simulink model "dsa2k_iwave_ospfb_4800"  (R2021a)
settings: Solver=VariableStepAuto  StartTime=0.0  StopTime=10.0  RelTol=1e-3
undefined symbols (not defined in the file): datetime, i, posixtime
libraries: xbsIndex_r4 x6279, casper_library_misc x96, casper_library_reorder x16, casper_library_delays x16, casper_library_accumulators x7, xps_library x3
(part 1 of 75)
settings Model: Creator=jackh  LastModifiedBy=jackh

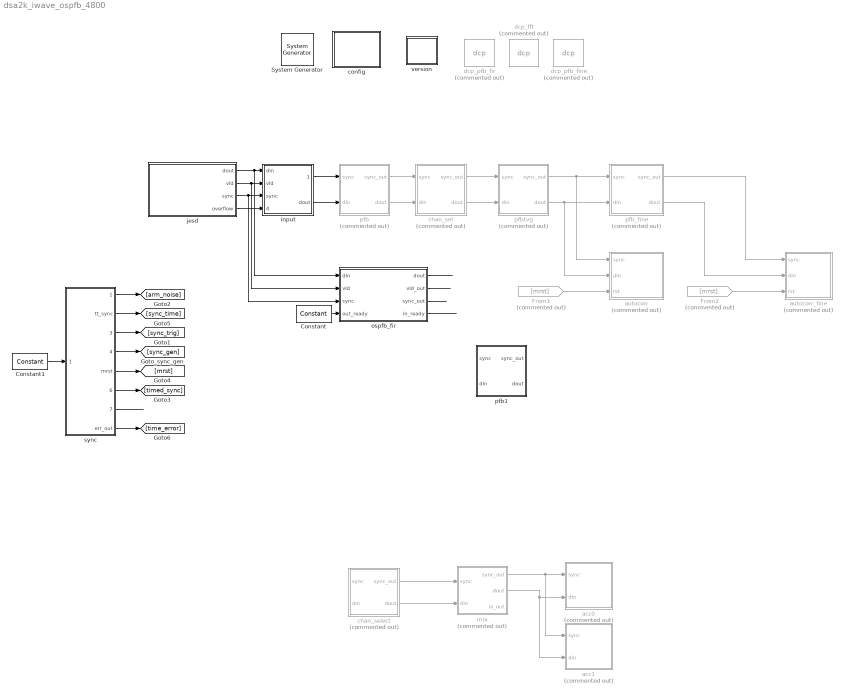
== system dsa2k_iwave_ospfb_4800 ==
  " System Generator" : xbsIndex_r4/ System Generator  Tag=genX  xilinxfamily=zynquplus  part=xczu11eg  speed=-1-i  package=ffvc1760  synthesis_tool=XST  clock_wrapper=Clock Enables  directory=/home/jackh/src/dsa2000-fpga/firmware/src/models/dsa2k_iwave_ospfb_4800/sysgen  proj_type=Vivado  Synth_file=Vivado Synthesis Defaults  Impl_file=Vivado Implementation Defaults  testbench=off  simulink_period=1  sysclk_period=3.3333  dcm_input_clock_period=10  incr_netlist=off  trim_vbits=Everywhere in SubSystem  dbl_ovrd=According to Block Masks  core_generation=According to Block Masks  run_coregen=off  deprecated_control=off  eval_field=0  block_type=sysgen
  Constant : xbsIndex_r4/Constant  const=1.0  gui_display_data_type=Boolean  arith_type=Boolean  n_bits=16  bin_pt=14  preci_type=Single  exp_width=8  frac_width=24  explicit_period=on  period=1  equ=P=C  opselect=C  inp2=PCIN>>17  opr=+  inp1=P  carry=CIN  dbl_ovrd=off  block_type=constant
  Constant1 : xbsIndex_r4/Constant  const=0  gui_display_data_type=Boolean  arith_type=Boolean  n_bits=16  bin_pt=14  preci_type=Single  exp_width=8  frac_width=24  explicit_period=on  period=1  equ=P=C  opselect=C  inp2=PCIN>>17  opr=+  inp1=P  carry=CIN  dbl_ovrd=off  block_type=constant
  From1 : From  Commented=on  GotoTag=mrst
  From2 : From  Commented=on  GotoTag=mrst
  acc0 : Subsystem  Commented=on  mask{nchan_serial_bits=8}
      mask prompts: nchan_serial_bits "Number of serial channels (2^?)"
  acc1 : Subsystem  Commented=on  mask{nchan_serial_bits=8}
      mask prompts: nchan_serial_bits "Number of serial channels (2^?)"
  autocorr : Subsystem  Commented=on  mask{nchan_bits=10-3, npol_bits=0}
      mask prompts: nchan_bits "Number of *SERIAL* channels (2^?)"; npol_bits "Number of pols (2^?)"
  autocorr_fine : Subsystem  Commented=on  mask{nchan_bits=14-3, npol_bits=0}
      mask prompts: nchan_bits "Number of *SERIAL* channels (2^?)"; npol_bits "Number of pols (2^?)"
  chan_sel : Subsystem  Commented=on
  chan_select : Subsystem  Commented=on  mask{serial_chan_bits=8}
      mask prompts: serial_chan_bits "Number of serial channels (2^?)"
  config : Subsystem  Tag=xps:xsg  mask(xsg core config){hw_sys=iwave_zu11:xczu11eg, clk_src=dsp_clk, clk_rate=4800/16 * 4 / 3, no_block_diagram=on, sample_period=1, synthesis_tool=XST}
      mask prompts: hw_sys "Hardware Platform"; clk_src "User IP Clock source"; clk_rate "User IP Clock Rate (MHz)"; no_block_diagram "Skip inclusion of infrastructure block diagram"; sample_period "Sample Period"; synthesis_tool "Synthesis Tool:"
      mask help:
      | The XSG Core Config block is used to configure the System Generator design
      | for the casper_xps toolflow. Settings here are used to configure the
      | Xilinx System Generator block parameters automatically, and control toolflow
      | script  execution. It needs to be at the top level of all designs being compiled
      | with the casper_xps toolflow.
      mask init:
      | xps_xsg_iwave_zu11_conf_mask;
      mask Help: eval('xlWeb([getenv(''MLIB_ROOT''), ''\doc\html\sys_xsg_core_config\sys_xsg_core_config.html''])')
      mask TypeOptions hw_sys: iwave_zu11:xczu11eg
      mask TypeOptions clk_src: sys_clk | adc_clk | clk300mhz | dsp_clk
      mask TypeOptions synthesis_tool: Leonardo Spectrum | Synplify | Synplify Pro | XST
      mask Display: fprintf(['iWave_ZU11']);
  dcp_fft : xps_library/Utilities/dcp  Tag=xps:dcp  Commented=on  dcp_file=[fileparts(which(bdroot)) '/dsp/fft_2p_4kc_18i_18o_core/fft_2p_4kc_18i_18o_core.dcp']
      settings: SourceProductName=CASPER XPS Blockset
  dcp_pfb_fine : xps_library/Utilities/dcp  Tag=xps:dcp  Commented=on  dcp_file=[fileparts(which(bdroot)) '/dsp/pfb_fine_core/pfb_fine_core.dcp']
      settings: SourceProductName=CASPER XPS Blockset
  dcp_pfb_fir : xps_library/Utilities/dcp  Tag=xps:dcp  Commented=on  dcp_file=[fileparts(which(bdroot)) '/dsp/pfb_fir_2p_2kpt_12i_18o_os2_core/pfb_fir_2p_2kpt_12i_18o_os2_core.dcp']
      settings: SourceProductName=CASPER XPS Blockset
  input : Subsystem
  jesd : Subsystem  Tag=xps:adi_jesd  mask(xsg_adi_jesd){fmc_port=0, adi_ip_path=/home/jackh/src/dsa2000-fpga/firmware/lib/adi_hdl/library, sample_rate_mhz=4800}
      mask prompts: fmc_port "FMC Port Number"; adi_ip_path "Path to ADI IP repository"; sample_rate_mhz "Sample rate (Msps)"
      mask init:
      | adi_jesd_init()
      mask Help: eval('xlWeb([getenv(''MLIB_ROOT''), ''\doc\html\sys_xsg_core_config\sys_xsg_core_config.html''])')
  mix : Subsystem  Commented=on  mask{serial_chan_bits=8}
      mask prompts: serial_chan_bits "Number of serial channels (2^?)"
  ospfb_fir : Subsystem  Tag=xps:ospfb_fir  mask(xsg_ospfb_fir){constants_path=[fileparts(which(bdroot)) '/config'], coeffs_path=[fileparts(which(bdroot)) '/config'], samples_per_clock=16}
      mask prompts: constants_path "Directory containing alpaca_constants_pkg.sv"; coeffs_path "Directory containing alpaca_ospfb_hann_2048_8_coeff_pkg.sv"; samples_per_clock "Parallel samples per clock"
      mask init:
      | ospfb_fir_init()
      mask Help: eval('xlWeb([getenv(''MLIB_ROOT''), ''\doc\html\sys_xsg_core_config\sys_xsg_core_config.html''])')
  pfb : Subsystem  Commented=on
  pfb1 : Subsystem
  pfb_fine : Subsystem  Commented=on
  pfbtvg : Subsystem  Commented=on  mask{serial_chan_bits=8}
      mask prompts: serial_chan_bits "Serial channels (2^?)"
  sync : Subsystem  mask{sync_lsb_bits=14, sync_period=12800000}
      mask prompts: sync_lsb_bits "Allowed sync granularity (2^?)"; sync_period "Expected_sync_period"
  version : Subsystem  mask{fw_type=2, ver_maj=1, ver_min=0, ver_rev=0, ver_bugfix=0}
      mask prompts: fw_type "Firmware Type"; ver_maj "Major version"; ver_min "Minor version"; ver_rev "Revision"; ver_bugfix "Bugfix"
  wires:
  sync/1(arm_noise) -> [arm_noise]
  sync/2(tt_sync) -> [sync_time]
  sync/5(mrst) -> [mrst]
  sync/3(ext_sync) -> [sync_trig]
  sync/6(timed_sync) -> [timed_sync]
  sync/4(sync_out) -> [sync_gen]
  sync/8(err_out) -> [time_error]
  sync/7(tt_int_out) -> ?
  Constant1/1 -> sync/1(sync_in)
  input/1(sync_out) -> pfb/1(sync)
  input/2(dout) -> pfb/2(din)
  pfbtvg/1(sync_out) -> pfb_fine/1(sync), autocorr/1(sync)
  chan_select/1(sync_out) -> mix/1(sync)
  chan_select/2(dout) -> mix/2(din)
  mix/1(sync_out) -> acc1/1(sync), acc0/1(sync)
  mix/2(dout) -> acc1/2(din), acc0/2(din)
  From1/1 -> autocorr/3(rst)
  jesd/2(vld) -> ospfb_fir/2(vld), input/2(vld)
  jesd/3(sync) -> ospfb_fir/3(sync), input/3(sync)
  jesd/4(overflow) -> input/4(overflow)
  jesd/1(dout) -> ospfb_fir/1(din), input/1(din)
  pfbtvg/2(dout) -> pfb_fine/2(din), autocorr/2(din)
  pfb_fine/2(dout) -> autocorr_fine/2(din)
  From2/1 -> autocorr_fine/3(rst)
  pfb_fine/1(sync_out) -> autocorr_fine/1(sync)
  pfb/1(sync_out) -> chan_sel/1(sync)
  pfb/2(dout) -> chan_sel/2(din)
  chan_sel/1(sync_out) -> pfbtvg/1(sync)
  chan_sel/2(dout) -> pfbtvg/2(din)
  Constant/1 -> ospfb_fir/4(out_ready)
  ospfb_fir/1(dout) -> ?
  ospfb_fir/2(vld_out) -> ?
  ospfb_fir/3(sync_out) -> ?
  ospfb_fir/4(in_ready) -> ?

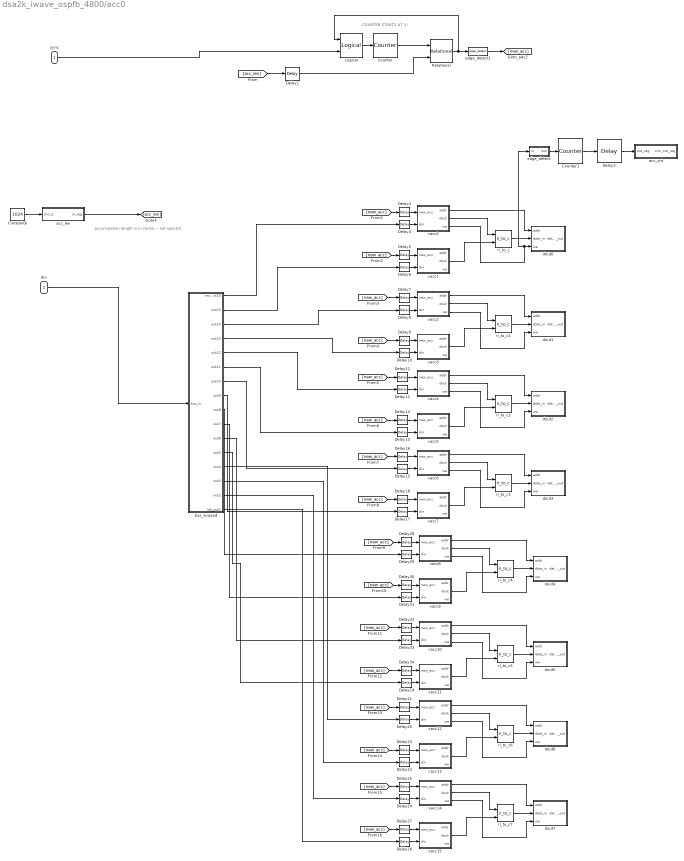
== system dsa2k_iwave_ospfb_4800/acc0 ==
  note: COUNTER STARTS AT 1!
  note: accumulation length is in clocks -- not spectra
  sync : Inport
  din : Inport  Port=2
  Constant6 : Constant  Value=1024
  Counter : xbsIndex_r4/Counter  cnt_type=Free Running  cnt_to=Inf  operation=Up  start_count=1  cnt_by_val=1  arith_type=Unsigned  n_bits=32  bin_pt=0  load_pin=off  rst=on  en=off  explicit_period=on  period=1  use_behavioral_HDL=on  implementation=Fabric  dbl_ovrd=off  block_type=counter
  Counter1 : xbsIndex_r4/Counter  cnt_type=Free Running  cnt_to=Inf  operation=Up  start_count=0  cnt_by_val=1  arith_type=Unsigned  n_bits=32  bin_pt=0  load_pin=off  rst=off  en=on  explicit_period=on  period=1  use_behavioral_HDL=on  implementation=Fabric  dbl_ovrd=off  block_type=counter
  Delay{1..34} (34 alike) : xbsIndex_r4/Delay  rst=off  infoeditControl=Selection of Reset will increase slice count due to use of real FFs and instead of SRLs  en=off  latency=1  reg_retiming=on  dbl_ovrd=off  block_type=delay
  Logical : xbsIndex_r4/Logical  logical_function=OR  inputs=2  en=off  latency=0  precision=Full  arith_type=Unsigned  n_bits=16  bin_pt=0  align_bp=on  dbl_ovrd=off  block_type=logical
  Relational : xbsIndex_r4/Relational  mode=a=b  op_type=Bool  en=off  latency=0  dbl_ovrd=off  block_type=relational
  acc_cnt : Subsystem  Tag=xps:sw_reg  AncestorBlock=xps_library/Memory/software_register  mask(swreg){io_dir=To Processor, io_delay=0, init_val=0, sample_period=1, names=reg, bitwidths=32, bin_pts=0, arith_types=0, sim_port=on, show_format=on, desc_str=|}
      mask desc_str=|
      | 32-bit wrapping accumulation counter, which increments each
      | time a new accumulation is recorded to RAM.
      | There is no buffer locking when correlation data are
      | read, so this counter can be used to ensure that data
      | have not changed during a read.
      mask prompts: io_dir "I/O direction"; io_delay "I/O delay"; init_val "Initial Value"; sample_period "Sample period"; names "Bitfield names [msb...lsb]"; bitwidths "Bitfield widths"; bin_pts "Bitfield binary pts"; arith_types "Bitfield types, ufix=0, fix=1, bool=2"; sim_port "Provide sim input/output?"; show_format "Print format string?"; desc_str "Description"
      mask help: A 32-bit software-accessible register. Can be divided into bitfields of varying widths and types using the fields in the block mask.
      mask init:
      | swreg_init(gcb)
      settings: AttributesFormatString=1output:uf32.0 = 32 bits
      mask TypeOptions io_dir: To Processor | From Processor
      mask Callback io_dir:
      | mask_enables = get_param(gcb, 'MaskEnables');
      | mask_names = get_param(gcb, 'MaskNames');
      | if strcmp(get_param(gcb, 'io_dir'), 'To Processor'),
      |     mask_enables{ismember(mask_names, 'sample_period')} = 'off';
      | else
      |     mask_enables{ismember(mask_names, 'sample_period')} = 'on';
      | end
      | set_param(gcb, 'MaskEnables', mask_enables);
      mask DialogControl ParameterTabVar0 Prompt: Setup
  acc_len : Subsystem  Tag=xps:sw_reg  AncestorBlock=xps_library/Memory/software_register  mask(swreg){io_dir=From Processor, io_delay=0, init_val=0, sample_period=1, names=reg, bitwidths=32, bin_pts=0, arith_types=0, sim_port=on, show_format=on, desc_str=|}
      mask desc_str=|
      | Accumulation length, in FPGA clock cycles. To specify
      | an accumulation length as a number of spectra this
      | register should be written with ``number_of_spectra x
      | frequency_channels_per_spectra``. Here the number
      | of frequency channels per spectra is the number
      | *output* by the correlation subsystem.
      | Glitches may occur (resulting in the no new
      | accumulations for a few seconds) if the value in this
      | register is reduced without re-applying a sync to the
      | correlation module.
      mask prompts: io_dir "I/O direction"; io_delay "I/O delay"; init_val "Initial Value"; sample_period "Sample period"; names "Bitfield names [msb...lsb]"; bitwidths "Bitfield widths"; bin_pts "Bitfield binary pts"; arith_types "Bitfield types, ufix=0, fix=1, bool=2"; sim_port "Provide sim input/output?"; show_format "Print format string?"; desc_str "Description"
      mask help: A 32-bit software-accessible register. Can be divided into bitfields of varying widths and types using the fields in the block mask.
      mask init:
      | swreg_init(gcb)
      settings: AttributesFormatString=1input:uf32.0 = 32 bits
      mask TypeOptions io_dir: To Processor | From Processor
      mask Callback io_dir:
      | mask_enables = get_param(gcb, 'MaskEnables');
      | mask_names = get_param(gcb, 'MaskNames');
      | if strcmp(get_param(gcb, 'io_dir'), 'To Processor'),
      |     mask_enables{ismember(mask_names, 'sample_period')} = 'off';
      | else
      |     mask_enables{ismember(mask_names, 'sample_period')} = 'on';
      | end
      | set_param(gcb, 'MaskEnables', mask_enables);
      mask DialogControl ParameterTabVar0 Prompt: Setup
  bus_expand : Subsystem  AncestorBlock=casper_library_flow_control/bus_expand  mask(bus_expand){mode=divisions of equal size, outputNum=16, outputWidth=20, outputBinaryPt=18, outputArithmeticType=1, show_format=off, outputToWorkspace=off, variablePrefix=out, outputToModelAsWell=on}
      mask prompts: outputNum "Number of outputs:"; outputWidth "Output width:"; outputBinaryPt "Output binary point position:"; outputArithmeticType "Output arithmetic type (ufix=0, fix=1, bool=2):"; show_format "Print format string?"; outputToWorkspace "Output to workspace?"; variablePrefix "Variable name prefix:"; outputToModelAsWell "Output to model as well?"
      mask help:
      | Expands a 'bus' made using a bus_create or Xilinx
      | concat block.
      | The input will be divided into the specified number
      | of outputs with the specified arithmetic types.
      | Divisions are made from most significant bit.
      mask init:
      | bus_expand_init(gcb,...
      |     'mode', mode, ...
      |     'outputNum', outputNum, ...
      |     'outputWidth', outputWidth, ...
      |     'outputBinaryPt', outputBinaryPt, ...
      |     'outputArithmeticType', outputArithmeticType, ...
      |     'show_format', show_format, ...
      |     'outputToWorkspace', outputToWorkspace, ...
      |     'variablePrefix', variablePrefix, ...
      |     'outputToModelAsWell', outputToModelAsWell);
      settings: AttributesFormatString=16 outputs
      mask TypeOptions mode: divisions of equal size | divisions of arbitrary size
      mask Callback mode: %bus_expand_callback();
      mask Callback outputWidth: %bus_expand_callback();
      mask Callback outputToWorkspace: %bus_expand_callback();
  dout0 : Subsystem  Tag=xps:bram  AncestorBlock=xps_library/Memory/shared_bram  mask{sample_rate=1, init_vals=[0:2^10-1], data_bin_pt=0, optimization=Minimum_Area, reg_core_output=off, reg_prim_output=off, data_width=64, addr_width=nchan_serial_bits, arith_type=Unsigned, desc_str=|, type_desc=uint64}
      mask desc_str=|
      | Correlation data buffer. Word ``[2n]`` is the
      | real part of the correlation of frequency channel ``n``
      | (after any channel averaging). Word ``[2n+1]`` is
      | the imaginary part of this correlation.
      mask prompts: sample_rate "Sample rate"; init_vals "Initial values (simulation only)"; data_bin_pt "Data Binary Point"; reg_core_output "Register Core Output"; reg_prim_output "Register Primitive Output"; data_width "Data Width"; addr_width "Address width"; arith_type "Output Data Type"; desc_str "Description"; type_desc "Word Type Description"
      mask init:
      | shared_bram_mask;
      mask TypeOptions optimization: Minimum_Area | Low_Power
      mask TypeOptions data_width: 8 | 16 | 32 | 64 | 128
      mask TypeOptions arith_type: Unsigned | Signed  (2's comp)
      mask DialogControl Container4 Prompt: Configuration
      mask DialogControl Container10 Prompt: Documentation
  dout1 : Subsystem  Tag=xps:bram  AncestorBlock=xps_library/Memory/shared_bram  mask{sample_rate=1, init_vals=[0:2^10-1], data_bin_pt=0, optimization=Minimum_Area, reg_core_output=off, reg_prim_output=off, data_width=64, addr_width=nchan_serial_bits, arith_type=Unsigned, desc_str=|, type_desc=uint64}
      mask desc_str=|
      | Correlation data buffer. Word ``[2n]`` is the
      | real part of the correlation of frequency channel ``n``
      | (after any channel averaging). Word ``[2n+1]`` is
      | the imaginary part of this correlation.
      mask prompts: sample_rate "Sample rate"; init_vals "Initial values (simulation only)"; data_bin_pt "Data Binary Point"; reg_core_output "Register Core Output"; reg_prim_output "Register Primitive Output"; data_width "Data Width"; addr_width "Address width"; arith_type "Output Data Type"; desc_str "Description"; type_desc "Word Type Description"
      mask init:
      | shared_bram_mask;
      mask TypeOptions optimization: Minimum_Area | Low_Power
      mask TypeOptions data_width: 8 | 16 | 32 | 64 | 128
      mask TypeOptions arith_type: Unsigned | Signed  (2's comp)
      mask DialogControl Container4 Prompt: Configuration
      mask DialogControl Container10 Prompt: Documentation
  dout2 : Subsystem  Tag=xps:bram  AncestorBlock=xps_library/Memory/shared_bram  mask{sample_rate=1, init_vals=[0:2^10-1], data_bin_pt=0, optimization=Minimum_Area, reg_core_output=off, reg_prim_output=off, data_width=64, addr_width=nchan_serial_bits, arith_type=Unsigned, desc_str=|, type_desc=uint64}
      mask desc_str=|
      | Correlation data buffer. Word ``[2n]`` is the
      | real part of the correlation of frequency channel ``n``
      | (after any channel averaging). Word ``[2n+1]`` is
      | the imaginary part of this correlation.
      mask prompts: sample_rate "Sample rate"; init_vals "Initial values (simulation only)"; data_bin_pt "Data Binary Point"; reg_core_output "Register Core Output"; reg_prim_output "Register Primitive Output"; data_width "Data Width"; addr_width "Address width"; arith_type "Output Data Type"; desc_str "Description"; type_desc "Word Type Description"
      mask init:
      | shared_bram_mask;
      mask TypeOptions optimization: Minimum_Area | Low_Power
      mask TypeOptions data_width: 8 | 16 | 32 | 64 | 128
      mask TypeOptions arith_type: Unsigned | Signed  (2's comp)
      mask DialogControl Container4 Prompt: Configuration
      mask DialogControl Container10 Prompt: Documentation
  dout3 : Subsystem  Tag=xps:bram  AncestorBlock=xps_library/Memory/shared_bram  mask{sample_rate=1, init_vals=[0:2^10-1], data_bin_pt=0, optimization=Minimum_Area, reg_core_output=off, reg_prim_output=off, data_width=64, addr_width=nchan_serial_bits, arith_type=Unsigned, desc_str=|, type_desc=uint64}
      mask desc_str=|
      | Correlation data buffer. Word ``[2n]`` is the
      | real part of the correlation of frequency channel ``n``
      | (after any channel averaging). Word ``[2n+1]`` is
      | the imaginary part of this correlation.
      mask prompts: sample_rate "Sample rate"; init_vals "Initial values (simulation only)"; data_bin_pt "Data Binary Point"; reg_core_output "Register Core Output"; reg_prim_output "Register Primitive Output"; data_width "Data Width"; addr_width "Address width"; arith_type "Output Data Type"; desc_str "Description"; type_desc "Word Type Description"
      mask init:
      | shared_bram_mask;
      mask TypeOptions optimization: Minimum_Area | Low_Power
      mask TypeOptions data_width: 8 | 16 | 32 | 64 | 128
      mask TypeOptions arith_type: Unsigned | Signed  (2's comp)
      mask DialogControl Container4 Prompt: Configuration
      mask DialogControl Container10 Prompt: Documentation
  dout4 : Subsystem  Tag=xps:bram  AncestorBlock=xps_library/Memory/shared_bram  mask{sample_rate=1, init_vals=[0:2^10-1], data_bin_pt=0, optimization=Minimum_Area, reg_core_output=off, reg_prim_output=off, data_width=64, addr_width=nchan_serial_bits, arith_type=Unsigned, desc_str=|, type_desc=uint64}
      mask desc_str=|
      | Correlation data buffer. Word ``[2n]`` is the
      | real part of the correlation of frequency channel ``n``
      | (after any channel averaging). Word ``[2n+1]`` is
      | the imaginary part of this correlation.
      mask prompts: sample_rate "Sample rate"; init_vals "Initial values (simulation only)"; data_bin_pt "Data Binary Point"; reg_core_output "Register Core Output"; reg_prim_output "Register Primitive Output"; data_width "Data Width"; addr_width "Address width"; arith_type "Output Data Type"; desc_str "Description"; type_desc "Word Type Description"
      mask init:
      | shared_bram_mask;
      mask TypeOptions optimization: Minimum_Area | Low_Power
      mask TypeOptions data_width: 8 | 16 | 32 | 64 | 128
      mask TypeOptions arith_type: Unsigned | Signed  (2's comp)
      mask DialogControl Container4 Prompt: Configuration
      mask DialogControl Container10 Prompt: Documentation
  dout5 : Subsystem  Tag=xps:bram  AncestorBlock=xps_library/Memory/shared_bram  mask{sample_rate=1, init_vals=[0:2^10-1], data_bin_pt=0, optimization=Minimum_Area, reg_core_output=off, reg_prim_output=off, data_width=64, addr_width=nchan_serial_bits, arith_type=Unsigned, desc_str=|, type_desc=uint64}
      mask desc_str=|
      | Correlation data buffer. Word ``[2n]`` is the
      | real part of the correlation of frequency channel ``n``
      | (after any channel averaging). Word ``[2n+1]`` is
      | the imaginary part of this correlation.
      mask prompts: sample_rate "Sample rate"; init_vals "Initial values (simulation only)"; data_bin_pt "Data Binary Point"; reg_core_output "Register Core Output"; reg_prim_output "Register Primitive Output"; data_width "Data Width"; addr_width "Address width"; arith_type "Output Data Type"; desc_str "Description"; type_desc "Word Type Description"
      mask init:
      | shared_bram_mask;
      mask TypeOptions optimization: Minimum_Area | Low_Power
      mask TypeOptions data_width: 8 | 16 | 32 | 64 | 128
      mask TypeOptions arith_type: Unsigned | Signed  (2's comp)
      mask DialogControl Container4 Prompt: Configuration
      mask DialogControl Container10 Prompt: Documentation
  dout6 : Subsystem  Tag=xps:bram  AncestorBlock=xps_library/Memory/shared_bram  mask{sample_rate=1, init_vals=[0:2^10-1], data_bin_pt=0, optimization=Minimum_Area, reg_core_output=off, reg_prim_output=off, data_width=64, addr_width=nchan_serial_bits, arith_type=Unsigned, desc_str=|, type_desc=uint64}
      mask desc_str=|
      | Correlation data buffer. Word ``[2n]`` is the
      | real part of the correlation of frequency channel ``n``
      | (after any channel averaging). Word ``[2n+1]`` is
      | the imaginary part of this correlation.
      mask prompts: sample_rate "Sample rate"; init_vals "Initial values (simulation only)"; data_bin_pt "Data Binary Point"; reg_core_output "Register Core Output"; reg_prim_output "Register Primitive Output"; data_width "Data Width"; addr_width "Address width"; arith_type "Output Data Type"; desc_str "Description"; type_desc "Word Type Description"
      mask init:
      | shared_bram_mask;
      mask TypeOptions optimization: Minimum_Area | Low_Power
      mask TypeOptions data_width: 8 | 16 | 32 | 64 | 128
      mask TypeOptions arith_type: Unsigned | Signed  (2's comp)
      mask DialogControl Container4 Prompt: Configuration
      mask DialogControl Container10 Prompt: Documentation
  dout7 : Subsystem  Tag=xps:bram  AncestorBlock=xps_library/Memory/shared_bram  mask{sample_rate=1, init_vals=[0:2^10-1], data_bin_pt=0, optimization=Minimum_Area, reg_core_output=off, reg_prim_output=off, data_width=64, addr_width=nchan_serial_bits, arith_type=Unsigned, desc_str=|, type_desc=uint64}
      mask desc_str=|
      | Correlation data buffer. Word ``[2n]`` is the
      | real part of the correlation of frequency channel ``n``
      | (after any channel averaging). Word ``[2n+1]`` is
      | the imaginary part of this correlation.
      mask prompts: sample_rate "Sample rate"; init_vals "Initial values (simulation only)"; data_bin_pt "Data Binary Point"; reg_core_output "Register Core Output"; reg_prim_output "Register Primitive Output"; data_width "Data Width"; addr_width "Address width"; arith_type "Output Data Type"; desc_str "Description"; type_desc "Word Type Description"
      mask init:
      | shared_bram_mask;
      mask TypeOptions optimization: Minimum_Area | Low_Power
      mask TypeOptions data_width: 8 | 16 | 32 | 64 | 128
      mask TypeOptions arith_type: Unsigned | Signed  (2's comp)
      mask DialogControl Container4 Prompt: Configuration
      mask DialogControl Container10 Prompt: Documentation
  edge_detect : Subsystem  AncestorBlock=casper_library_misc/edge_detect  mask(edge_detect){edge=Falling, polarity=Active High, x_in=[0 0.08 0.08 0.16 0.16 0.24 0.24 0.32 0.32 0.4], y_in=[-1 -1  1  1  1  1  1  1  1  1], x_out=[0.6 0.68 0.68 0.76 0.76 0.84 0.84 0.92 0.92 1], y_out=[-1 -1  1  1 -1 -1 -1 -1 -1 -1]}
      mask prompts: edge "Edge Type"; polarity "Output Polarity"; x_in "Input X Positions"; y_in "Input Y Positions"; x_out "Output X Positions"; y_out "Output Y Positions"
      mask help: Output is active for one-cycle after each edge of the specified type (i.e. rising, falling or both).
      mask init:
      | edge_detect_init(gcb,...
      |     'edge',edge,...
      |     'polarity',polarity,...
      |     'x_in',x_in,...
      |     'x_out',x_out,...
      |     'y_in',y_in,...
      |     'y_out',y_out);
      | 
      | x_in_num=str2num(getfield(getfield(get_param(gcb,'UserData'),'parameters'),'x_in'));
      | x_out_num=str2num(getfield(getfield(get_param(gcb,'UserData'),'parameters'),'x_out'));
      | y_in_num=str2num(getfield(getfield(get_param(gcb,'UserData'),'parameters'),'y_in'));
      | y_out_num=str2num(getfield(getfield(get_param(gcb,'UserData'),'parameters'),'y_out'));
      settings: AttributesFormatString=|
      | falling edges
      | active high
      mask Help: Output is active for one-cycle after each edge of the specified type (i.e. rising, falling, or both).  Latency is zero.
      mask TypeOptions edge: Rising | Falling | Both
      mask TypeOptions polarity: Active High | Active Low
      mask Display:
      | plot(x_in_num,0.5+y_in_num*0.2);
      | plot(x_out_num,0.5+y_out_num*0.2);
  edge_detect1 : casper_library_misc/edge_detect  edge=Rising  polarity=Active High  x_in=[0 0.08 0.08 0.16 0.16 0.24 0.24 0.32 0.32 0.4]  y_in="[-1 -1  1  1  1  1  1  1  1  1]"  x_out=[0.6 0.68 0.68 0.76 0.76 0.84 0.84 0.92 0.92 1]  y_out="[-1 -1  1  1 -1 -1 -1 -1 -1 -1]"
  ri_to_c{,1..7} (8 alike) : casper_library_misc/ri_to_c
      settings: SourceProductName=CASPER DSP Blockset
  vacc0 : Subsystem  AncestorBlock=casper_library_accumulators/addr_bram_vacc  mask(simple_bram_vacc){vec_len=2^(nchan_serial_bits), arith_type=Signed, n_bits=32, bin_pt=18}
      mask prompts: vec_len "Vector length:"; arith_type "Output type:"; n_bits "Bit width (output):"; bin_pt "Binary point (output):"
      mask help: This simple vector accumulator is based on a shift register. It outputs its previous accumulated vector after a new_acc pulse is received.
      mask init:
      | simple_bram_vacc_init(gcb, ...
      |     'vec_len', vec_len, ...
      |     'arith_type', arith_type, ...
      |     'n_bits', n_bits, ...
      |     'bin_pt', bin_pt);
      mask TypeOptions arith_type: Signed | Unsigned
  vacc1 : Subsystem  AncestorBlock=casper_library_accumulators/addr_bram_vacc  mask(simple_bram_vacc){vec_len=2^(nchan_serial_bits), arith_type=Signed, n_bits=32, bin_pt=18}
      mask prompts: vec_len "Vector length:"; arith_type "Output type:"; n_bits "Bit width (output):"; bin_pt "Binary point (output):"
      mask help: This simple vector accumulator is based on a shift register. It outputs its previous accumulated vector after a new_acc pulse is received.
      mask init:
      | simple_bram_vacc_init(gcb, ...
      |     'vec_len', vec_len, ...
      |     'arith_type', arith_type, ...
      |     'n_bits', n_bits, ...
      |     'bin_pt', bin_pt);
      mask TypeOptions arith_type: Signed | Unsigned
  vacc10 : Subsystem  AncestorBlock=casper_library_accumulators/addr_bram_vacc  mask(simple_bram_vacc){vec_len=2^(nchan_serial_bits), arith_type=Signed, n_bits=32, bin_pt=18}
      mask prompts: vec_len "Vector length:"; arith_type "Output type:"; n_bits "Bit width (output):"; bin_pt "Binary point (output):"
      mask help: This simple vector accumulator is based on a shift register. It outputs its previous accumulated vector after a new_acc pulse is received.
      mask init:
      | simple_bram_vacc_init(gcb, ...
      |     'vec_len', vec_len, ...
      |     'arith_type', arith_type, ...
      |     'n_bits', n_bits, ...
      |     'bin_pt', bin_pt);
      mask TypeOptions arith_type: Signed | Unsigned
  vacc11 : Subsystem  AncestorBlock=casper_library_accumulators/addr_bram_vacc  mask(simple_bram_vacc){vec_len=2^(nchan_serial_bits), arith_type=Signed, n_bits=32, bin_pt=18}
      mask prompts: vec_len "Vector length:"; arith_type "Output type:"; n_bits "Bit width (output):"; bin_pt "Binary point (output):"
      mask help: This simple vector accumulator is based on a shift register. It outputs its previous accumulated vector after a new_acc pulse is received.
      mask init:
      | simple_bram_vacc_init(gcb, ...
      |     'vec_len', vec_len, ...
      |     'arith_type', arith_type, ...
      |     'n_bits', n_bits, ...
      |     'bin_pt', bin_pt);
      mask TypeOptions arith_type: Signed | Unsigned
  vacc12 : Subsystem  AncestorBlock=casper_library_accumulators/addr_bram_vacc  mask(simple_bram_vacc){vec_len=2^(nchan_serial_bits), arith_type=Signed, n_bits=32, bin_pt=18}
      mask prompts: vec_len "Vector length:"; arith_type "Output type:"; n_bits "Bit width (output):"; bin_pt "Binary point (output):"
      mask help: This simple vector accumulator is based on a shift register. It outputs its previous accumulated vector after a new_acc pulse is received.
      mask init:
      | simple_bram_vacc_init(gcb, ...
      |     'vec_len', vec_len, ...
      |     'arith_type', arith_type, ...
      |     'n_bits', n_bits, ...
      |     'bin_pt', bin_pt);
      mask TypeOptions arith_type: Signed | Unsigned
  vacc13 : Subsystem  AncestorBlock=casper_library_accumulators/addr_bram_vacc  mask(simple_bram_vacc){vec_len=2^(nchan_serial_bits), arith_type=Signed, n_bits=32, bin_pt=18}
      mask prompts: vec_len "Vector length:"; arith_type "Output type:"; n_bits "Bit width (output):"; bin_pt "Binary point (output):"
      mask help: This simple vector accumulator is based on a shift register. It outputs its previous accumulated vector after a new_acc pulse is received.
      mask init:
      | simple_bram_vacc_init(gcb, ...
      |     'vec_len', vec_len, ...
      |     'arith_type', arith_type, ...
      |     'n_bits', n_bits, ...
      |     'bin_pt', bin_pt);
      mask TypeOptions arith_type: Signed | Unsigned
  vacc14 : Subsystem  AncestorBlock=casper_library_accumulators/addr_bram_vacc  mask(simple_bram_vacc){vec_len=2^(nchan_serial_bits), arith_type=Signed, n_bits=32, bin_pt=18}
      mask prompts: vec_len "Vector length:"; arith_type "Output type:"; n_bits "Bit width (output):"; bin_pt "Binary point (output):"
      mask help: This simple vector accumulator is based on a shift register. It outputs its previous accumulated vector after a new_acc pulse is received.
      mask init:
      | simple_bram_vacc_init(gcb, ...
      |     'vec_len', vec_len, ...
      |     'arith_type', arith_type, ...
      |     'n_bits', n_bits, ...
      |     'bin_pt', bin_pt);
      mask TypeOptions arith_type: Signed | Unsigned
  vacc15 : Subsystem  AncestorBlock=casper_library_accumulators/addr_bram_vacc  mask(simple_bram_vacc){vec_len=2^(nchan_serial_bits), arith_type=Signed, n_bits=32, bin_pt=18}
      mask prompts: vec_len "Vector length:"; arith_type "Output type:"; n_bits "Bit width (output):"; bin_pt "Binary point (output):"
      mask help: This simple vector accumulator is based on a shift register. It outputs its previous accumulated vector after a new_acc pulse is received.
      mask init:
      | simple_bram_vacc_init(gcb, ...
      |     'vec_len', vec_len, ...
      |     'arith_type', arith_type, ...
      |     'n_bits', n_bits, ...
      |     'bin_pt', bin_pt);
      mask TypeOptions arith_type: Signed | Unsigned
  vacc2 : Subsystem  AncestorBlock=casper_library_accumulators/addr_bram_vacc  mask(simple_bram_vacc){vec_len=2^(nchan_serial_bits), arith_type=Signed, n_bits=32, bin_pt=18}
      mask prompts: vec_len "Vector length:"; arith_type "Output type:"; n_bits "Bit width (output):"; bin_pt "Binary point (output):"
      mask help: This simple vector accumulator is based on a shift register. It outputs its previous accumulated vector after a new_acc pulse is received.
      mask init:
      | simple_bram_vacc_init(gcb, ...
      |     'vec_len', vec_len, ...
      |     'arith_type', arith_type, ...
      |     'n_bits', n_bits, ...
      |     'bin_pt', bin_pt);
      mask TypeOptions arith_type: Signed | Unsigned
  vacc3 : Subsystem  AncestorBlock=casper_library_accumulators/addr_bram_vacc  mask(simple_bram_vacc){vec_len=2^(nchan_serial_bits), arith_type=Signed, n_bits=32, bin_pt=18}
      mask prompts: vec_len "Vector length:"; arith_type "Output type:"; n_bits "Bit width (output):"; bin_pt "Binary point (output):"
      mask help: This simple vector accumulator is based on a shift register. It outputs its previous accumulated vector after a new_acc pulse is received.
      mask init:
      | simple_bram_vacc_init(gcb, ...
      |     'vec_len', vec_len, ...
      |     'arith_type', arith_type, ...
      |     'n_bits', n_bits, ...
      |     'bin_pt', bin_pt);
      mask TypeOptions arith_type: Signed | Unsigned
  vacc4 : Subsystem  AncestorBlock=casper_library_accumulators/addr_bram_vacc  mask(simple_bram_vacc){vec_len=2^(nchan_serial_bits), arith_type=Signed, n_bits=32, bin_pt=18}
      mask prompts: vec_len "Vector length:"; arith_type "Output type:"; n_bits "Bit width (output):"; bin_pt "Binary point (output):"
      mask help: This simple vector accumulator is based on a shift register. It outputs its previous accumulated vector after a new_acc pulse is received.
      mask init:
      | simple_bram_vacc_init(gcb, ...
      |     'vec_len', vec_len, ...
      |     'arith_type', arith_type, ...
      |     'n_bits', n_bits, ...
      |     'bin_pt', bin_pt);
      mask TypeOptions arith_type: Signed | Unsigned
  vacc5 : Subsystem  AncestorBlock=casper_library_accumulators/addr_bram_vacc  mask(simple_bram_vacc){vec_len=2^(nchan_serial_bits), arith_type=Signed, n_bits=32, bin_pt=18}
      mask prompts: vec_len "Vector length:"; arith_type "Output type:"; n_bits "Bit width (output):"; bin_pt "Binary point (output):"
      mask help: This simple vector accumulator is based on a shift register. It outputs its previous accumulated vector after a new_acc pulse is received.
      mask init:
      | simple_bram_vacc_init(gcb, ...
      |     'vec_len', vec_len, ...
      |     'arith_type', arith_type, ...
      |     'n_bits', n_bits, ...
      |     'bin_pt', bin_pt);
      mask TypeOptions arith_type: Signed | Unsigned
  vacc6 : Subsystem  AncestorBlock=casper_library_accumulators/addr_bram_vacc  mask(simple_bram_vacc){vec_len=2^(nchan_serial_bits), arith_type=Signed, n_bits=32, bin_pt=18}
      mask prompts: vec_len "Vector length:"; arith_type "Output type:"; n_bits "Bit width (output):"; bin_pt "Binary point (output):"
      mask help: This simple vector accumulator is based on a shift register. It outputs its previous accumulated vector after a new_acc pulse is received.
      mask init:
      | simple_bram_vacc_init(gcb, ...
      |     'vec_len', vec_len, ...
      |     'arith_type', arith_type, ...
      |     'n_bits', n_bits, ...
      |     'bin_pt', bin_pt);
      mask TypeOptions arith_type: Signed | Unsigned
  vacc7 : Subsystem  AncestorBlock=casper_library_accumulators/addr_bram_vacc  mask(simple_bram_vacc){vec_len=2^(nchan_serial_bits), arith_type=Signed, n_bits=32, bin_pt=18}
      mask prompts: vec_len "Vector length:"; arith_type "Output type:"; n_bits "Bit width (output):"; bin_pt "Binary point (output):"
      mask help: This simple vector accumulator is based on a shift register. It outputs its previous accumulated vector after a new_acc pulse is received.
      mask init:
      | simple_bram_vacc_init(gcb, ...
      |     'vec_len', vec_len, ...
      |     'arith_type', arith_type, ...
      |     'n_bits', n_bits, ...
      |     'bin_pt', bin_pt);
      mask TypeOptions arith_type: Signed | Unsigned
  vacc8 : Subsystem  AncestorBlock=casper_library_accumulators/addr_bram_vacc  mask(simple_bram_vacc){vec_len=2^(nchan_serial_bits), arith_type=Signed, n_bits=32, bin_pt=18}
      mask prompts: vec_len "Vector length:"; arith_type "Output type:"; n_bits "Bit width (output):"; bin_pt "Binary point (output):"
      mask help: This simple vector accumulator is based on a shift register. It outputs its previous accumulated vector after a new_acc pulse is received.
      mask init:
      | simple_bram_vacc_init(gcb, ...
      |     'vec_len', vec_len, ...
      |     'arith_type', arith_type, ...
      |     'n_bits', n_bits, ...
      |     'bin_pt', bin_pt);
      mask TypeOptions arith_type: Signed | Unsigned
  vacc9 : Subsystem  AncestorBlock=casper_library_accumulators/addr_bram_vacc  mask(simple_bram_vacc){vec_len=2^(nchan_serial_bits), arith_type=Signed, n_bits=32, bin_pt=18}
      mask prompts: vec_len "Vector length:"; arith_type "Output type:"; n_bits "Bit width (output):"; bin_pt "Binary point (output):"
      mask help: This simple vector accumulator is based on a shift register. It outputs its previous accumulated vector after a new_acc pulse is received.
      mask init:
      | simple_bram_vacc_init(gcb, ...
      |     'vec_len', vec_len, ...
      |     'arith_type', arith_type, ...
      |     'n_bits', n_bits, ...
      |     'bin_pt', bin_pt);
      mask TypeOptions arith_type: Signed | Unsigned
  wires:
  din/1 -> bus_expand/1(bus_in)
  Counter1/1 -> Delay2/1
  edge_detect/1(out) -> Counter1/1
  acc_len/1(in_reg) -> [acc_len]
  vacc0/2(dout) -> ri_to_c/1
  Constant6/1 -> acc_len/1(sim_1)
  Logical/1 -> Counter/1
  ri_to_c/1 -> dout0/2(data_in)
  vacc1/2(dout) -> ri_to_c/2
  Relational/1 -> edge_detect1/1, Logical/1
  Delay2/1 -> acc_cnt/1(out_reg)
  [acc_len] -> Delay1/1
  vacc0/3(we) -> dout0/3(we), edge_detect/1(in)
  vacc0/1(addr) -> dout0/1(addr)
  vacc2/1(addr) -> dout1/1(addr)
  vacc2/3(we) -> dout1/3(we)
  vacc3/2(dout) -> ri_to_c1/2
  ri_to_c1/1 -> dout1/2(data_in)
  vacc2/2(dout) -> ri_to_c1/1
  vacc4/2(dout) -> ri_to_c2/1
  ri_to_c2/1 -> dout2/2(data_in)
  vacc5/2(dout) -> ri_to_c2/2
  vacc4/3(we) -> dout2/3(we)
  vacc4/1(addr) -> dout2/1(addr)
  vacc6/1(addr) -> dout3/1(addr)
  vacc6/3(we) -> dout3/3(we)
  vacc7/2(dout) -> ri_to_c3/2
  ri_to_c3/1 -> dout3/2(data_in)
  vacc6/2(dout) -> ri_to_c3/1
  bus_expand/8(out9) -> Delay17/1
  bus_expand/1(msb_out16) -> Delay4/1
  bus_expand/2(out15) -> Delay6/1
  bus_expand/3(out14) -> Delay8/1
  bus_expand/4(out13) -> Delay10/1
  bus_expand/5(out12) -> Delay11/1
  bus_expand/6(out11) -> Delay13/1
  bus_expand/7(out10) -> Delay15/1
  Counter/1 -> Relational/1
  edge_detect1/1 -> [new_acc]
  [new_acc] -> Delay3/1
  [new_acc] -> Delay5/1
  [new_acc] -> Delay7/1
  [new_acc] -> Delay9/1
  [new_acc] -> Delay12/1
  [new_acc] -> Delay14/1
  [new_acc] -> Delay16/1
  [new_acc] -> Delay18/1
  Delay1/1 -> Relational/2
  Delay3/1 -> vacc0/1(new_acc)
  Delay4/1 -> vacc0/2(din)
  Delay5/1 -> vacc1/1(new_acc)
  Delay6/1 -> vacc1/2(din)
  Delay7/1 -> vacc2/1(new_acc)
  Delay8/1 -> vacc2/2(din)
  Delay10/1 -> vacc3/2(din)
  Delay9/1 -> vacc3/1(new_acc)
  Delay12/1 -> vacc4/1(new_acc)
  Delay11/1 -> vacc4/2(din)
  Delay13/1 -> vacc5/2(din)
  Delay14/1 -> vacc5/1(new_acc)
  Delay16/1 -> vacc6/1(new_acc)
  Delay15/1 -> vacc6/2(din)
  Delay17/1 -> vacc7/2(din)
  Delay18/1 -> vacc7/1(new_acc)
  Delay27/1 -> vacc15/1(new_acc)
  Delay26/1 -> vacc15/2(din)
  Delay24/1 -> vacc14/2(din)
  Delay25/1 -> vacc14/1(new_acc)
  Delay23/1 -> vacc13/1(new_acc)
  Delay22/1 -> vacc13/2(din)
  Delay20/1 -> vacc12/2(din)
  Delay21/1 -> vacc12/1(new_acc)
  Delay34/1 -> vacc11/1(new_acc)
  Delay19/1 -> vacc11/2(din)
  Delay33/1 -> vacc10/2(din)
  Delay32/1 -> vacc10/1(new_acc)
  Delay31/1 -> vacc9/2(din)
  Delay30/1 -> vacc9/1(new_acc)
  Delay29/1 -> vacc8/2(din)
  Delay28/1 -> vacc8/1(new_acc)
  [new_acc] -> Delay27/1
  [new_acc] -> Delay25/1
  [new_acc] -> Delay23/1
  [new_acc] -> Delay21/1
  [new_acc] -> Delay34/1
  [new_acc] -> Delay32/1
  [new_acc] -> Delay30/1
  [new_acc] -> Delay28/1
  bus_expand/15(out2) -> Delay24/1
  bus_expand/14(out3) -> Delay22/1
  bus_expand/13(out4) -> Delay20/1
  bus_expand/12(out5) -> Delay19/1
  bus_expand/11(out6) -> Delay33/1
  bus_expand/10(out7) -> Delay31/1
  bus_expand/9(out8) -> Delay29/1
  bus_expand/16(lsb_out1) -> Delay26/1
  vacc14/2(dout) -> ri_to_c7/1
  ri_to_c7/1 -> dout7/2(data_in)
  vacc15/2(dout) -> ri_to_c7/2
  vacc14/3(we) -> dout7/3(we)
  vacc14/1(addr) -> dout7/1(addr)
  vacc12/1(addr) -> dout6/1(addr)
  vacc12/3(we) -> dout6/3(we)
  vacc13/2(dout) -> ri_to_c6/2
  ri_to_c6/1 -> dout6/2(data_in)
  vacc12/2(dout) -> ri_to_c6/1
  vacc10/2(dout) -> ri_to_c5/1
  ri_to_c5/1 -> dout5/2(data_in)
  vacc11/2(dout) -> ri_to_c5/2
  vacc10/3(we) -> dout5/3(we)
  vacc10/1(addr) -> dout5/1(addr)
  vacc8/1(addr) -> dout4/1(addr)
  vacc8/3(we) -> dout4/3(we)
  vacc9/2(dout) -> ri_to_c4/2
  ri_to_c4/1 -> dout4/2(data_in)
  vacc8/2(dout) -> ri_to_c4/1
  sync/1 -> Logical/2
